simulink model "lab1_2"  (R2016b)
settings: Solver=VariableStepAuto  StartTime=0.0  StopTime=10.0  RelTol=1e-3
libraries: simulink x2
settings Model: Creator=Emanuel  LastModifiedBy=Emanuel

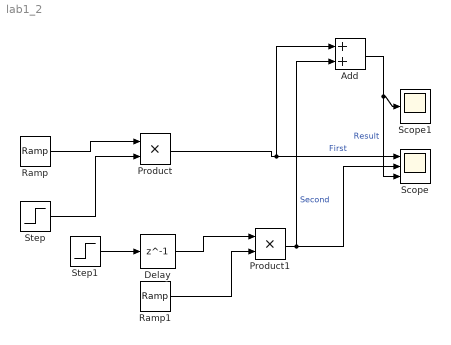
== system lab1_2 ==
  Add : Sum
  Delay : Delay  DelayLength=1  InitialCondition=0  SampleTime=1
  Product : Product
  Product1 : Product
  Ramp : simulink/Sources/Ramp  slope=1  start=0  X0=0
  Ramp1 : simulink/Sources/Ramp  slope=-1  start=1  X0=1
  Scope : Scope  NumInputPorts=3
  Scope1 : Scope
  Step : Step  Before=1  After=0  SampleTime=1
  Step1 : Step  Before=1  After=0  SampleTime=1
  wires:
  Ramp/1 -> Product/1
  Step/1 -> Product/2
  Product/1 -> Add/1, Scope/1  "First"
  Ramp1/1 -> Product1/2
  Product1/1 -> Add/2, Scope/2  "Second"
  Step1/1 -> Delay/1
  Delay/1 -> Product1/1
  Add/1 -> Scope1/1, Scope/3  "Result"
